simulink model "Op_Space_Impedance_Control"  (R2020b)
settings: Solver=VariableStepAuto  StartTime=0.0  StopTime=tk(end)-tk(1)  RelTol=1e-3
values from neighbouring files (symbols this model uses):
  B = myRobot.B_Lagrangian    [hw12_main.m]
  C = myRobot.C_Lagrangian    [hw12_main.m]
  dJ = myRobot.dJa    [hw12_main.m]
  F = myRobot.F    [hw12_main.m]
  G = myRobot.G_Lagrangian    [hw12_main.m]
  J = myRobot.J    [hw12_main.m]
  Ja = myRobot.Ja    [hw12_main.m]
  K = diag([1,100,10,1,1,1])    [hw12_main.m]
  Kd = diag([1,8,1,1,1,1]).*10    [hw12_main.m]
  Kp = diag([10,100,10,1,1,1]).*10    [hw12_main.m]
  Md = diag([1 1 1 0 0 0])    [hw12_main.m]
  Md_inv = pinv(Md)    [hw12_main.m]
  Ts = 0.001    [hw12_main.m]
  x_r = [0.2;0.26; 0.2502; -pi/2; -pi/2; -pi/2]    [hw12_main.m]
settings Model: Creator=nicol  LastModifiedBy=nicol
settings DebuggingCC: UnderSpecifiedDimensionMsg=warning

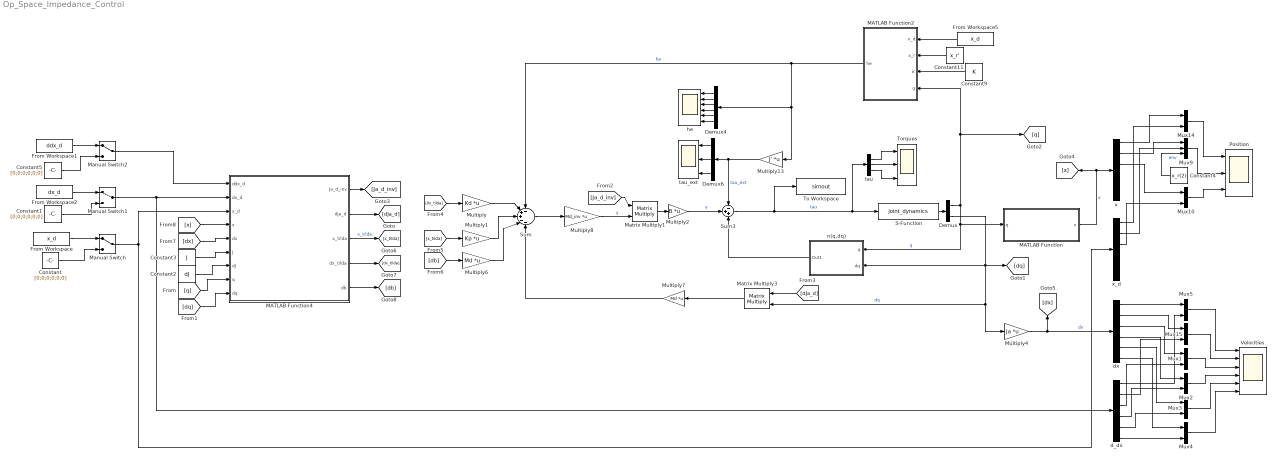
== system Op_Space_Impedance_Control ==
  Constant : Constant  Value=[0;0;0;0;0;0]
  Constant1 : Constant  Value=[0;0;0;0;0;0]
  Constant11 : Constant  Value=x_r'
  Constant2 : Constant  Value=dJ
  Constant3 : Constant  Value=J
  Constant4 : Constant  Value=x_r(2)
  Constant5 : Constant  Value=[0;0;0;0;0;0]
  Constant9 : Constant  Value=K
  Demux : Demux  Outputs=2
  Demux4 : Demux  Outputs=6
  Demux6 : Demux  Outputs=3
  From Workspace : FromWorkspace  VariableName=x_d  SampleTime=Ts
  From Workspace1 : FromWorkspace  VariableName=ddx_d  SampleTime=Ts
  From Workspace2 : FromWorkspace  VariableName=dx_d  SampleTime=Ts
  From Workspace5 : FromWorkspace  VariableName=x_d  SampleTime=Ts
  MATLAB Function : MATLAB Function  TreatAsAtomicUnit=on
  MATLAB Function2 : MATLAB Function  TreatAsAtomicUnit=on
  MATLAB Function4 : MATLAB Function  TreatAsAtomicUnit=on
  Manual Switch : ManualSwitch
  Manual Switch1 : ManualSwitch
  Manual Switch2 : ManualSwitch
  Matrix Multiply1 : Product  Multiplication=Matrix(*)
  Matrix Multiply3 : Product  Multiplication=Matrix(*)
  Multiply : Gain  Gain=Kd  Multiplication=Matrix(K*u)
  Multiply1 : Gain  Gain=Kp  Multiplication=Matrix(K*u)
  Multiply13 : Gain  Gain=J'  Multiplication=Matrix(K*u)
  Multiply2 : Gain  Gain=B  Multiplication=Matrix(K*u)
  Multiply4 : Gain  Gain=Ja  Multiplication=Matrix(K*u)
  Multiply6 : Gain  Gain=Md  Multiplication=Matrix(K*u)
  Multiply7 : Gain  Gain=Md  Multiplication=Matrix(K*u)
  Multiply8 : Gain  Gain=Md_inv  Multiplication=Matrix(K*u)
  Mux{1..5,10,14..15} (8 alike) : Mux  Inputs=2
  Mux9 : Mux  Inputs=3
  Position : Scope  NumInputPorts=3
  S-Function : S-Function  FunctionName=joint_dynamics  Parameters=myRobot  SFunctionDeploymentMode=off  EnableBusSupport=off
  Sum : Sum  Inputs=-++--
  Sum3 : Sum  Inputs=-++
  To Workspace : ToWorkspace  VariableName=simout  SaveFormat=Timeseries  SampleTime=-1
  Torques : Scope  NumInputPorts=3
  Velocities : Scope  NumInputPorts=6
  d_dx : Demux  Outputs=6
  dx : Demux  Outputs=6
  he : Scope  NumInputPorts=6
  n(q,dq) : Subsystem
  tau : Demux  Outputs=3
  tau_ext : Scope  NumInputPorts=3
  x : Demux  Outputs=6
  x_d : Demux  Outputs=6
  wires:
  From Workspace2/1 -> Manual Switch1/1
  From Workspace/1 -> Manual Switch/1
  Sum3/1 -> To Workspace/1, S-Function/1, tau/1  "tau"
  S-Function/1 -> Demux/1
  Demux/2 -> n(q,dq)/2(dq), [dq], Multiply4/1, Matrix Multiply3/2  "dq"
  n(q,dq)/1(Out1) -> Sum3/3
  Constant1/1 -> Manual Switch1/2
  Manual Switch1/1 -> d_dx/1, MATLAB Function4/2(dx_d)
  tau/1 -> Torques/1
  tau/2 -> Torques/2
  Multiply4/1 -> dx/1, [dx]  "dx"
  Sum/1 -> Multiply8/1
  Multiply8/1 -> Matrix Multiply1/2  "y"
  x_d/2 -> Mux9/2
  Mux14/1 -> Position/1
  Mux10/1 -> Position/3
  x/3 -> Mux10/1
  x_d/1 -> Mux14/2
  x_d/3 -> Mux10/2
  Mux9/1 -> Position/2
  x/1 -> Mux14/1
  d_dx/1 -> Mux5/2
  dx/1 -> Mux5/1
  Mux5/1 -> Velocities/1
  dx/5 -> Mux3/1
  Mux3/1 -> Velocities/5
  d_dx/4 -> Mux2/2
  d_dx/6 -> Mux4/2
  dx/4 -> Mux2/1
  d_dx/3 -> Mux1/2
  d_dx/2 -> Mux15/2
  d_dx/5 -> Mux3/2
  Mux15/1 -> Velocities/2
  dx/3 -> Mux1/1
  Mux2/1 -> Velocities/4
  dx/2 -> Mux15/1
  dx/6 -> Mux4/1
  Mux4/1 -> Velocities/6
  Mux1/1 -> Velocities/3
  Matrix Multiply3/1 -> Multiply7/1
  Demux4/6 -> he/6
  Demux4/5 -> he/5
  Demux4/2 -> he/2
  Demux4/4 -> he/4
  Demux4/3 -> he/3
  Demux4/1 -> he/1
  Demux6/1 -> tau_ext/1
  Demux6/2 -> tau_ext/2
  Demux6/3 -> tau_ext/3
  Multiply13/1 -> Sum3/1, Demux6/1  "tau_ext"
  tau/3 -> Torques/3
  [x_tilda] -> Multiply1/1
  [dx_tilda] -> Multiply/1
  [db] -> Multiply6/1
  Multiply/1 -> Sum/2
  Multiply1/1 -> Sum/3
  Multiply6/1 -> Sum/4
  [dJa_d] -> Matrix Multiply3/1
  Multiply7/1 -> Sum/5
  MATLAB Function/1(x) -> [x], x/1  "x"
  Matrix Multiply1/1 -> Multiply2/1
  Manual Switch/1 -> x_d/1, MATLAB Function4/3(x_d)
  [q] -> MATLAB Function4/8(q)
  Constant3/1 -> MATLAB Function4/6(J)
  MATLAB Function4/1(Ja_d_inv) -> [Ja_d_inv]
  MATLAB Function4/2(dJa_d) -> [dJa_d]
  [Ja_d_inv] -> Matrix Multiply1/1
  MATLAB Function4/3(x_tilda) -> [x_tilda]  "x_tilda"
  MATLAB Function4/4(dx_tilda) -> [dx_tilda]
  MATLAB Function4/5(db) -> [db]
  [dx] -> MATLAB Function4/5(dx)
  [x] -> MATLAB Function4/4(x)
  From Workspace1/1 -> Manual Switch2/1
  Manual Switch2/1 -> MATLAB Function4/1(ddx_d)
  [dq] -> MATLAB Function4/9(dq)
  Constant2/1 -> MATLAB Function4/7(dJ)
  x/2 -> Mux9/1
  Constant4/1 -> Mux9/3  "env"
  Constant/1 -> Manual Switch/2
  Constant5/1 -> Manual Switch2/2
  Multiply2/1 -> Sum3/2  "y"
  MATLAB Function2/1(he) -> Sum/1, Demux4/1, Multiply13/1  "he"
  From Workspace5/1 -> MATLAB Function2/1(x_d)
  Demux/1 -> MATLAB Function2/4(q), [q], n(q,dq)/1(q), MATLAB Function/1(q)  "q"
  Constant9/1 -> MATLAB Function2/3(K)
  Constant11/1 -> MATLAB Function2/2(x_r)

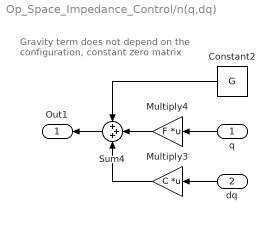
== system Op_Space_Impedance_Control/n(q,dq) ==
  note: Gravity term does not depend on the
      |  configuration, constant zero matrix
  q : Inport
  dq : Inport  Port=2
  Constant2 : Constant  Value=G  VectorParams1D=off
  Multiply3 : Gain  Gain=C  Multiplication=Matrix(K*u)
  Multiply4 : Gain  Gain=F  Multiplication=Matrix(K*u)
  Sum4 : Sum  Inputs=+++
  Out1 : Outport
  wires:
  Sum4/1 -> Out1/1
  Multiply3/1 -> Sum4/3
  Multiply4/1 -> Sum4/2
  Constant2/1 -> Sum4/1
  q/1 -> Multiply4/1
  dq/1 -> Multiply3/1

== matlab function Op_Space_Impedance_Control/MATLAB Function ==
  data: q input size=3; x output size=6
function x = directKinematics(q)
x=[ q(1) + 1/5;
    q(3) + 1/5;
    q(2) + 1251/5000;
    -pi/2;
    -pi/2;
    -pi/2];
end

== matlab function Op_Space_Impedance_Control/MATLAB Function2 ==
  data: x_d input; x_r input; K input; q input; he output
function he = Environment(x_d,x_r,K,q)

T_e=getTe(q);
x_e=zeros(6,1);
x_e(1:3,1)=T_e(1:3,4);
eul_e = rotm2eul(T_e(1:3,1:3),'ZYZ');
x_e(4:6,1)=eul_e;

if(x_e(2,1)-x_r(2,1)<0)
    he=[0;0;0;0;0;0];
else
    sup=zeros(6,1);
    dx_r_d=x_d-x_r;
    dx_e_d=x_d-x_e;
    sup(2,1)=dx_r_d(2,1)-dx_e_d(2,1);
    he=K*sup;
end

== matlab function Op_Space_Impedance_Control/MATLAB Function4 ==
  data: ddx_d input; dx_d input; x_d input; x input size=[6,1]; dx input; J input; dJ input; q input size=[3,1]; Ja_d_inv output size=[3,6]; dJa_d output size=[6,3]; x_tilda output size=[6,1]; dx_tilda output size=[6,1]; db output size=[6,1]; dq input size=[3,1]
function [Ja_d_inv,dJa_d,x_tilda,dx_tilda,db]=fnc(ddx_d,dx_d,x_d,x,dx,J,dJ,q,dq)
% desired rotational matrix
phi_d=x_d(4:6,1);
R_d=eul2rotm(phi_d','ZYZ');
T_d=[R_d, x_d(1:3); [0 0 0 1]];

% end effector rotational matrix
T_e=getTe(q);
R_e=T_e(1:3,1:3);

% COMPUTATION OF X_TILDA

% homogenous transf for end effector pose expressed in desired frame
T_e_d=pinv(T_d)*T_e;
R_e_d=T_e_d(1:3,1:3);
phi_e_d=rotm2eul(R_e_d,'ZYZ');
x_tilda=-[T_e_d(1:3,4);phi_e_d'];

Ta=getTa(phi_e_d(1),phi_e_d(2),phi_e_d(3));

Ta_inv=pinv(Ta);
% COMPUTATION OF JA_D, JA_D_INV

Ja_d=Ta_inv*[R_d', zeros(3);zeros(3), R_d']*J;
Ja_d_inv=zeros(3,6);
Ja_d_inv=pinv(Ja_d);

% COMPUTATION OF DX_TILDA

do_d=dx_d(1:3,1);
w_d=dx_d(4:6,1);
w_d_d=pinv(T_d)*[w_d;1];
w_d_d=w_d_d(1:3,1);
S=getS(w_d_d);
T=Ta(4:6,4:6);

% COMPUTATION OF B

b=[R_d'*do_d+S*x_tilda(1:3,1);
    pinv(T)*w_d_d];

dx_tilda=-Ja_d*dq+b;

% COMPUTATION OF DJA_D

w_d=dx_d(4:6,1);
S_w_d=getS(w_d);
dphi_e_d=pinv(Ta(4:6,4:6))*dx_d(4:6,1);
dTa=getDTa(phi_e_d(1),phi_e_d(2),phi_e_d(3),dphi_e_d(1),dphi_e_d(2),dphi_e_d(3));


first_term=Ta_inv*([R_d'*S_w_d,zeros(3,3);zeros(3,3),R_d'*S_w_d]*J + [R_d',zeros(3,3);zeros(3,3),R_d']*dJ);
dTa_inv=-Ta_inv*dTa*Ta_inv;
second_term=dTa_inv*[R_d',zeros(3,3);zeros(3,3),R_d']*J;
dJa_d = first_term+second_term;

% COMPUTATION OF DB

ddo_d=ddx_d(1:3,1);
dw_d=ddx_d(4:6,1);
o_d=x_d(1:3,1);
o_e=x(1:3,1);
do_e=dx(1:3,1);

firstTerm=R_d'*S_w_d*do_d + R_d'*ddo_d + R_d'*getS(dw_d)*(o_d-o_e) + R_d'*S_w_d*(do_d-do_e);

T_inv=pinv(T);
dT_inv=-T_inv*dTa(4:6,4:6)*T_inv;
secondTerm=dT_inv*R_d'*w_d + T_inv*R_d'*dw_d;

db=zeros(6,1);
db=[firstTerm;secondTerm];

end
